simulink model "GetSetParamExample"  (R2023b)
settings: Solver=VariableStepAuto  StartTime=0.0  StopTime=7e-2  MaxStep=1e-3  RelTol=1e-3
libraries: simulink x2
settings Model: Creator=rlschie  LastModifiedBy=rlschie

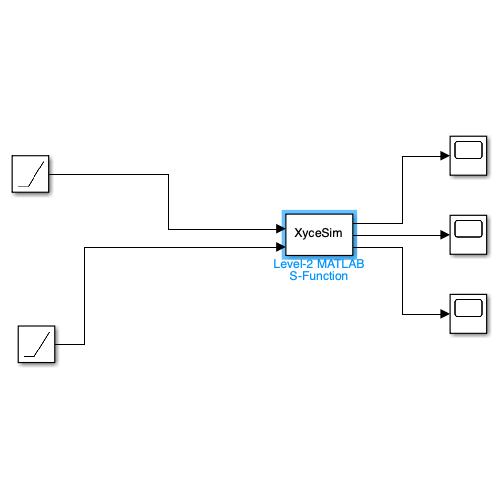
[thumbnail: Simulink's stored preview of the top-level diagram]
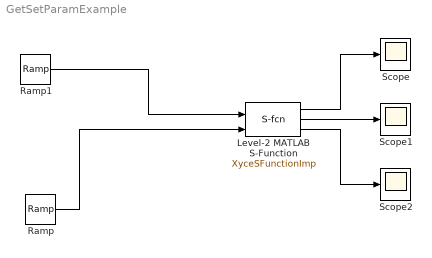
== system GetSetParamExample ==
  Level-2 MATLAB S-Function : M-S-Function  FunctionName=XyceSFunctionImp  Parameters=XyceInputFileName,WorkingDirectory,NumberOfInputs,NumberOfOutputs,InputNames,OutputNames  mask{XyceInputFileName=GetSetParams.cir, WorkingDirectory=/Users/rlschie/src/XyceDevelopment/INSTALL/share/SimulinkExamples/, XyceInputPortNames=, XyceOutputPortNames=, XyceNumberOfInputPorts=0, XyceNumberOfOutputPorts=0, NumberOfInputs=2, NumberOfOutputs=3, InputNames={ '1', 'TEMP'; '2', 'R1:R'; '-', '-' }, OutputNames={ '1', 'TEMP'; '2', 'R1:R'; '3', 'V(2)' }}
      mask prompts: XyceInputFileName "Xyce Input Filename"; WorkingDirectory "Working Directory"; XyceInputPortNames "Xyce Input Port Names"; XyceOutputPortNames "Xyce Output Port Names"; XyceNumberOfInputPorts "Xyce Number Of Inputs"; XyceNumberOfOutputPorts "Xyce Number Of Outputs"; NumberOfInputs "Number of Inputs"; NumberOfOutputs "Number of Outputs"; InputNames "Input Names"; OutputNames "Output Names"
      mask DialogControl SelectXyceInputFileButton Prompt: Select Xyce Input File
      mask DialogControl ScanXyceInputFileButton Prompt: Scan Xyce Input File
      mask DialogControl ResetForm Prompt: Reset
      mask Display: disp('XyceSim');
  Ramp : simulink/Sources/Ramp  slope=500  start=0  InitialOutput=100
  Ramp1 : simulink/Sources/Ramp  slope=-50  start=1e-3  InitialOutput=20
  Scope : Scope
  Scope1 : Scope
  Scope2 : Scope
  wires:
  Ramp1/1 -> Level-2 MATLAB S-Function/1
  Ramp/1 -> Level-2 MATLAB S-Function/2
  Level-2 MATLAB S-Function/1 -> Scope/1
  Level-2 MATLAB S-Function/2 -> Scope1/1
  Level-2 MATLAB S-Function/3 -> Scope2/1
